simulink model "yacc"  (R2020a)
settings: Solver=VariableStepAuto  StartTime=0.0  StopTime=10.0  RelTol=1e-3
undefined symbols (not defined in the file): Ay, m
settings Model: Creator=Muni Kumar  LastModifiedBy=Muni Kumar

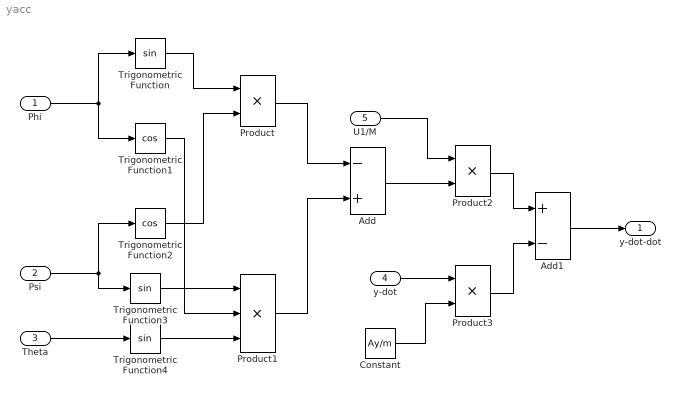
== system yacc ==
  Phi : Inport
  Psi : Inport  Port=2
  Theta : Inport  Port=3
  y-dot : Inport  Port=4
  U1/M : Inport  Port=5
  Add : Sum  Inputs=-+
  Add1 : Sum  Inputs=+-
  Constant : Constant  Value=Ay/m
  Product : Product
  Product1 : Product  Inputs=3
  Product2 : Product
  Product3 : Product
  Trigonometric Function : Trigonometry
  Trigonometric Function1 : Trigonometry  Operator=cos
  Trigonometric Function2 : Trigonometry  Operator=cos
  Trigonometric Function3 : Trigonometry
  Trigonometric Function4 : Trigonometry
  y-dot-dot : Outport
  wires:
  Product2/1 -> Add1/1
  Add/1 -> Product2/2
  Trigonometric Function/1 -> Product/1
  Add1/1 -> y-dot-dot/1
  Trigonometric Function3/1 -> Product1/1
  Phi/1 -> Trigonometric Function1/1, Trigonometric Function/1
  Theta/1 -> Trigonometric Function4/1
  Trigonometric Function2/1 -> Product/2
  Product/1 -> Add/1
  Product1/1 -> Add/2
  Psi/1 -> Trigonometric Function3/1, Trigonometric Function2/1
  Constant/1 -> Product3/2
  Product3/1 -> Add1/2
  Trigonometric Function4/1 -> Product1/3
  y-dot/1 -> Product3/1
  Trigonometric Function1/1 -> Product1/2
  U1/M/1 -> Product2/1
